simulink model "plant"  (R2021b)
settings: Solver=VariableStepAuto  StartTime=0.0  StopTime=100  RelTol=1e-3
model workspace (MAT data in the model file):
  M_k = 0.0296
  k_gear = 20.57
  length_init = 1
settings Model: Creator=bosto  LastModifiedBy=bosto

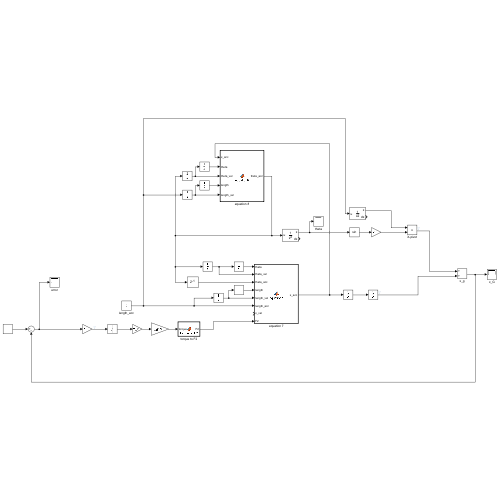
[thumbnail: Simulink's stored preview of the top-level diagram]
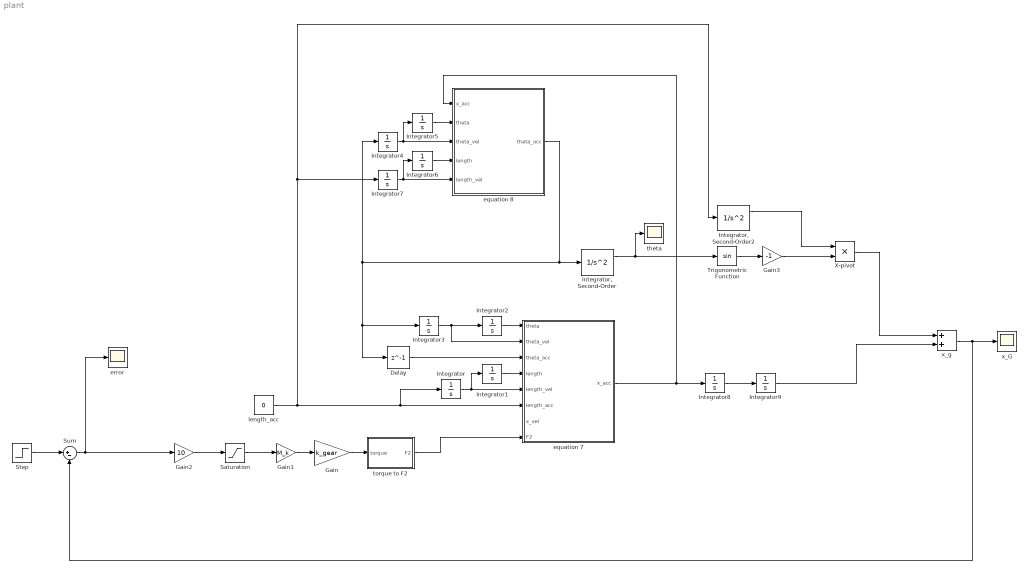
== system plant ==
  Delay : Delay  DelayLength=1  InitialCondition=0
  Gain : Gain  Gain=k_gear
  Gain1 : Gain  Gain=M_k
  Gain2 : Gain  Gain=10
  Gain3 : Gain  Gain=-1
  Integrator{,2..5,7..9} (8 alike) : Integrator
  "Integrator, Second-Order" : SecondOrderIntegrator
  "Integrator, Second-Order2" : SecondOrderIntegrator  ICX=length_init
  Integrator1 : Integrator  InitialCondition=length_init
  Integrator6 : Integrator  InitialCondition=length_init
  Saturation : Saturate  UpperLimit=10  LowerLimit=-10
  Step : Step  SampleTime=0
  Sum : Sum  Inputs=|+-
  Trigonometric Function : Trigonometry
  X-pivot : Product
  equation 7 : MATLAB Function  TreatAsAtomicUnit=on
  equation 8 : MATLAB Function  TreatAsAtomicUnit=on
  error : Scope
  length_acc : Constant  Value=0
  theta : Scope
  torque to F2 : MATLAB Function  TreatAsAtomicUnit=on
  x_G : Scope
  x_g : Sum
  wires:
  Integrator2/1 -> equation 7/1(theta)
  Integrator3/1 -> equation 7/2(theta_vel), Integrator2/1
  Integrator4/1 -> Integrator5/1, equation 8/3(theta_vel)
  Integrator5/1 -> equation 8/2(theta)
  Integrator/1 -> equation 7/5(length_vel), Integrator1/1
  Integrator1/1 -> equation 7/4(length)
  length_acc/1 -> Integrator7/1, "Integrator, Second-Order2"/1, Integrator/1, equation 7/6(length_acc)
  Integrator6/1 -> equation 8/4(length)
  Integrator7/1 -> Integrator6/1, equation 8/5(length_vel)
  "Integrator, Second-Order"/1 -> theta/1, Trigonometric Function/1
  equation 7/1(x_acc) -> Integrator8/1, equation 8/1(x_acc)
  Trigonometric Function/1 -> Gain3/1
  "Integrator, Second-Order2"/1 -> X-pivot/1
  X-pivot/1 -> x_g/1
  x_g/1 -> Sum/2, x_G/1
  torque to F2/1(F2) -> equation 7/8(F2)
  Step/1 -> Sum/1
  equation 8/1(theta_acc) -> Integrator4/1, Delay/1, Integrator3/1, "Integrator, Second-Order"/1
  Delay/1 -> equation 7/3(theta_acc)
  Gain/1 -> torque to F2/1(torque)
  Gain1/1 -> Gain/1
  Gain2/1 -> Saturation/1
  Saturation/1 -> Gain1/1
  Integrator8/1 -> Integrator9/1
  Integrator9/1 -> x_g/2
  Gain3/1 -> X-pivot/2
  Sum/1 -> Gain2/1, error/1

== matlab function plant/equation 8 ==
  data: x_acc input; theta_acc output; theta input; theta_vel input; length input; length_vel input
function theta_acc = equation8(x_acc, theta, theta_vel, length, length_vel)

theta_acc = -1/length * (2*length_vel*theta_vel + 9.82*sin(theta)+x_acc*cos(theta));

== matlab function plant/equation 7 ==
  data: theta input; theta_vel input; theta_acc input; length input; length_vel input; length_acc input; x_vel input; F2 input; x_acc output
function x_acc = equation7( theta, theta_vel, theta_acc, length, length_vel, length_acc, x_vel ,F2)
%todo, add dynamic friction

b1 = (3+1)/(3+1+.8+1.2e-3/.16^2);
Bd = 11;
x_radius = .16;
mC = 3;
mH = 1;
mT = .8;
I1 = 1.2e-3;



x_acc = F2;

x_acc = x_acc - b1*length_acc*sin(theta);

x_acc = x_acc- b1*length*theta_acc*cos(theta);

x_acc = x_acc + b1*length*theta_vel^2*sin(theta);

x_acc = x_acc + 2 * b1*length_vel*theta_vel*cos(theta);

x_acc = x_acc - x_vel*Bd/(mC+mH+mT + I1/x_radius^2);

== matlab function plant/torque to F2 ==
  data: torque input; F2 output
function F2 = torque_2_F2(torque)
x_radius = .16;
mC = 3;
mH = 1;
mT = .8;
I1 = 1.2e-3;

F2 = torque/x_radius/(mC+mH+mT + I1/x_radius^2);
